simulink model "SOC_Test"  (R2022b)
settings: Solver=VariableStepAuto  StartTime=0.0  StopTime=5100  RelTol=1e-3
values from neighbouring files (symbols this model uses):
  NumModules = 1.0    [Global_Parameters.sldd]
  NumParallel = 30.0    [Global_Parameters.sldd]
  NumSeries = 24.0    [Global_Parameters.sldd]
settings Model: DataDictionary=Global_Parameters.sldd  Creator=japerez  LastModifiedBy=japerez

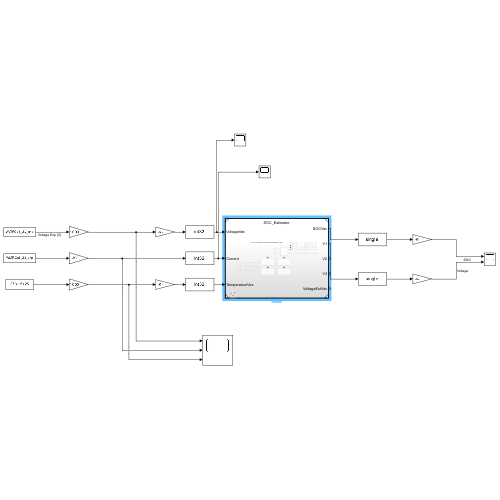
[thumbnail: Simulink's stored preview of the top-level diagram]
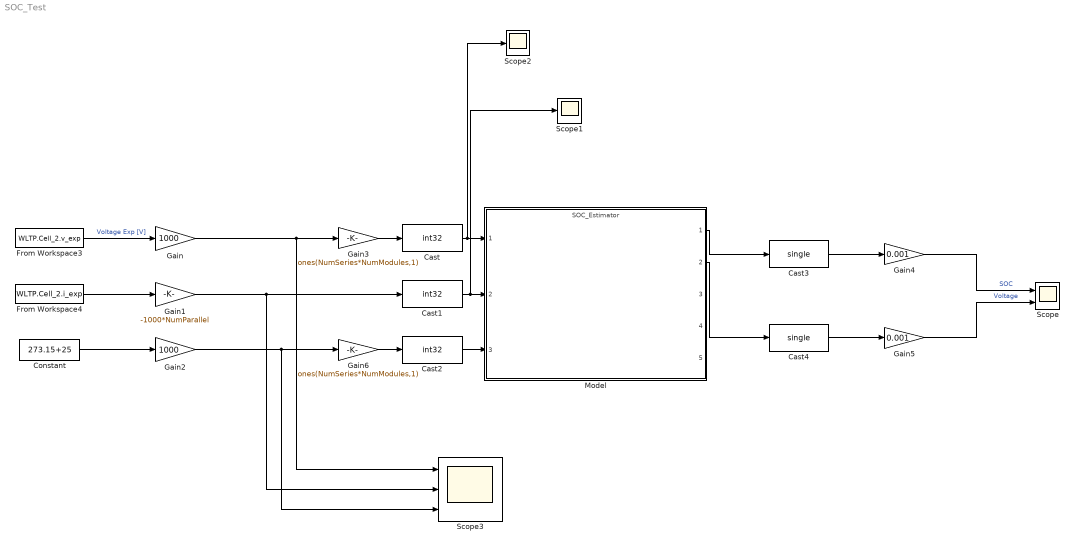
== system SOC_Test ==
  Cast : DataTypeConversion  OutDataTypeStr=int32  SaturateOnIntegerOverflow=off  RndMeth=Floor
  Cast1 : DataTypeConversion  OutDataTypeStr=int32  SaturateOnIntegerOverflow=off  RndMeth=Floor
  Cast2 : DataTypeConversion  OutDataTypeStr=int32  SaturateOnIntegerOverflow=off  RndMeth=Floor
  Cast3 : DataTypeConversion  OutDataTypeStr=single  SaturateOnIntegerOverflow=off  RndMeth=Floor
  Cast4 : DataTypeConversion  OutDataTypeStr=single  SaturateOnIntegerOverflow=off  RndMeth=Floor
  Constant : Constant  Value=273.15+25
  From Workspace3 : FromWorkspace  VariableName=WLTP.Cell_2.v_exp
  From Workspace4 : FromWorkspace  VariableName=WLTP.Cell_2.i_exp
  Gain : Gain  Gain=1000
  Gain1 : Gain  Gain=-1000*NumParallel
  Gain2 : Gain  Gain=1000
  Gain3 : Gain  Gain=ones(NumSeries*NumModules,1)
  Gain4 : Gain  Gain=0.001
  Gain5 : Gain  Gain=0.001
  Gain6 : Gain  Gain=ones(NumSeries*NumModules,1)
  Model : ModelReference  ModelNameDialog=SOC_Estimator.slx  SimulationMode=Normal  ModelReferenceVersion=1.31
  Scope : Scope  NumInputPorts=2
  Scope1 : Scope
  Scope2 : Scope
  Scope3 : Scope  NumInputPorts=3
  wires:
  From Workspace3/1 -> Gain/1  "Voltage Exp [V]"
  Gain/1 -> Scope3/1, Gain3/1
  Gain3/1 -> Cast/1
  From Workspace4/1 -> Gain1/1
  Cast/1 -> Scope2/1, Model/1
  Cast1/1 -> Scope1/1, Model/2
  Gain1/1 -> Scope3/2, Cast1/1
  Constant/1 -> Gain2/1
  Gain2/1 -> Scope3/3, Gain6/1
  Cast2/1 -> Model/3
  Model/1 -> Cast3/1
  Model/2 -> Cast4/1
  Cast3/1 -> Gain4/1
  Cast4/1 -> Gain5/1
  Gain4/1 -> Scope/1  "SOC"
  Gain5/1 -> Scope/2  "Voltage"
  Gain6/1 -> Cast2/1
